simulink model "NON_COHERENT_RECEIVER"  (R2021b)
settings: Solver=VariableStepAuto  StartTime=0.0  StopTime=inf  RelTol=1e-3
libraries: simulink x3, dspsigops x3, dsparch4 x2, commfilt2 x2, dspsrcs4 x1
settings Model: Creator=caccolillo  LastModifiedBy=caccolillo

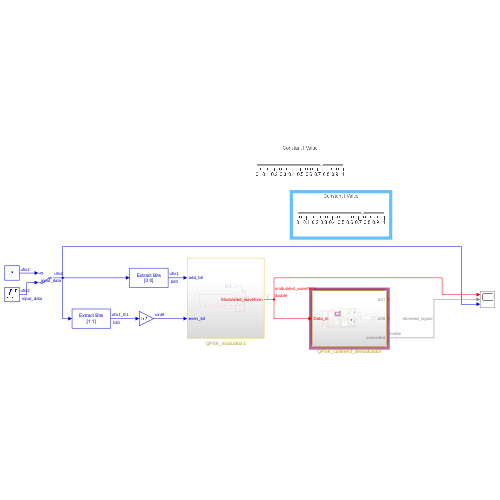
[thumbnail: Simulink's stored preview of the top-level diagram]
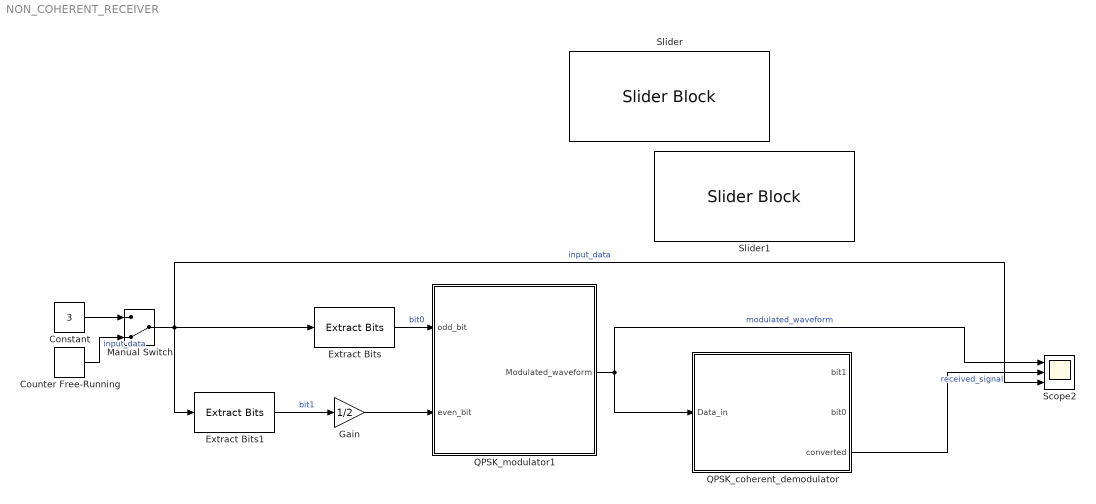
== system NON_COHERENT_RECEIVER ==
  Constant : Constant  Value=3  OutDataTypeStr=fixdt(0,2)  SampleTime=1/20000
  Counter Free-Running : simulink/Sources/Counter Free-Running  NumBits=2  tsamp=1/20000
  Extract Bits : simulink/Logic and Bit Operations/Extract Bits  bitsToExtract=Range of bits  numBits=8  bitIdxRange=[0 0]  outScalingMode=Preserve fixed-point scaling
  Extract Bits1 : simulink/Logic and Bit Operations/Extract Bits  bitsToExtract=Range of bits  numBits=8  bitIdxRange=[1 1]  outScalingMode=Preserve fixed-point scaling
  Gain : Gain  Gain=1/2
  Manual Switch : ManualSwitch  CurrentSetting=0
  QPSK_coherent_demodulator : Subsystem
  QPSK_modulator1 : Subsystem
  Scope2 : Scope  NumInputPorts=3
  Slider : SliderBlock  ScaleMax=1
  Slider1 : SliderBlock  ScaleMax=1
  wires:
  QPSK_modulator1/1(Modulated_waveform) -> QPSK_coherent_demodulator/1(Data_in), Scope2/1  "modulated_waveform"
  Manual Switch/1 -> Extract Bits1/1, Scope2/3, Extract Bits/1  "input_data"
  Gain/1 -> QPSK_modulator1/2(even_bit)
  Constant/1 -> Manual Switch/1
  Extract Bits1/1 -> Gain/1  "bit1"
  QPSK_coherent_demodulator/3(converted) -> Scope2/2  "received_signal"
  Counter Free-Running/1 -> Manual Switch/2  "input_data"
  Extract Bits/1 -> QPSK_modulator1/1(odd_bit)  "bit0"

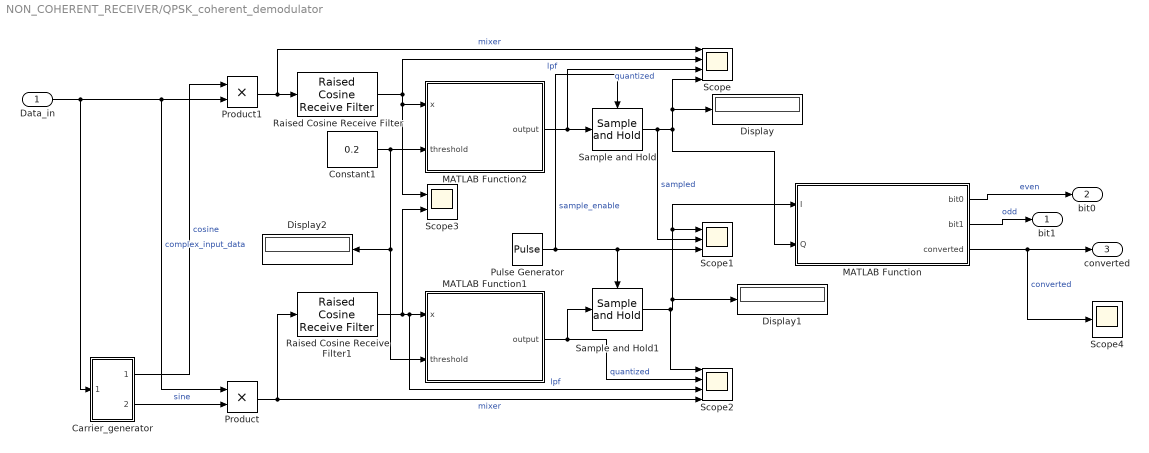
== system NON_COHERENT_RECEIVER/QPSK_coherent_demodulator ==
  Data_in : Inport
  Carrier_generator : Subsystem
  Constant1 : Constant  Value=0.2
  Display : Display
  Display1 : Display
  Display2 : Display
  MATLAB Function : MATLAB Function  TreatAsAtomicUnit=on
  MATLAB Function1 : MATLAB Function  TreatAsAtomicUnit=on
  MATLAB Function2 : MATLAB Function  TreatAsAtomicUnit=on
  Product : Product
  Product1 : Product
  Pulse Generator : DiscretePulseGenerator  PulseType=Time based  Period=1/20000  PulseWidth=5
  Raised Cosine Receive Filter : commfilt2/Raised Cosine Receive Filter  filtType=Square root  R=0.2  filtSpan=10  N=10  downFactor=2  downOffset=0  filterGain=1  RateOptions=Allow multirate processing  framing=Mute  checkCoeff=off  variableName=rcRxFilt  currentFiltSpan=10  D=5  inputOffset=0  sampMode=Mute  saveAsFlag=0  rateMode=Downsampling  checkGain=Normalized  launchFVT=on  roundingMode=Floor  overflowMode=off  coeffDataTypeStr=Inherit: Same word length as input  coeffMin=[]  coeffMax=[]  coeffLastDataTypeStr=Inherit: Same word length as input  accumDataTypeStr=Inherit: Same as product output  accumLastDataTypeStr=Inherit: Same as product output  outputDataTypeStr=Inherit: Same as accumulator  outputMin=[]  outputMax=[]  outputLastDataTypeStr=Inherit: Same as accumulator
  Raised Cosine Receive Filter1 : commfilt2/Raised Cosine Receive Filter  filtType=Square root  R=0.2  filtSpan=10  N=10  downFactor=2  downOffset=0  filterGain=1  RateOptions=Allow multirate processing  framing=Mute  checkCoeff=off  variableName=rcRxFilt1  currentFiltSpan=10  D=5  inputOffset=0  sampMode=Mute  saveAsFlag=0  rateMode=Downsampling  checkGain=Normalized  launchFVT=on  roundingMode=Floor  overflowMode=off  coeffDataTypeStr=Inherit: Same word length as input  coeffMin=[]  coeffMax=[]  coeffLastDataTypeStr=Inherit: Same word length as input  accumDataTypeStr=Inherit: Same as product output  accumLastDataTypeStr=Inherit: Same as product output  outputDataTypeStr=Inherit: Same as accumulator  outputMin=[]  outputMax=[]  outputLastDataTypeStr=Inherit: Same as accumulator
  Sample and Hold : dspsigops/Sample and Hold  trig=Rising edge  initCond=0  latchinput=off
  Sample and Hold1 : dspsigops/Sample and Hold  trig=Rising edge  initCond=0  latchinput=off
  Scope : Scope  NumInputPorts=4
  Scope1 : Scope  NumInputPorts=3
  Scope2 : Scope  NumInputPorts=4
  Scope3 : Scope  NumInputPorts=2
  Scope4 : Scope
  bit1 : Outport
  bit0 : Outport  Port=2
  converted : Outport  Port=3
  wires:
  Data_in/1 -> Carrier_generator/1(Modulated_signal), Product/1, Product1/2  "complex_input_data"
  Product1/1 -> Raised Cosine Receive Filter/1, Scope/1  "mixer"
  Raised Cosine Receive Filter/1 -> MATLAB Function2/1(x), Scope3/1, Scope/2  "lpf"
  Product/1 -> Raised Cosine Receive Filter1/1, Scope2/4  "mixer"
  Pulse Generator/1 -> Sample and Hold1/Trigger, Scope1/3, Sample and Hold/Trigger  "sample_enable"
  MATLAB Function1/1(output) -> Scope2/2, Sample and Hold1/1  "quantized"
  Sample and Hold/1 -> MATLAB Function/2(Q), Scope/4, Display/1, Scope1/2  "sampled"
  MATLAB Function2/1(output) -> Scope/3, Sample and Hold/1  "quantized"
  Carrier_generator/2(sine) -> Product/2  "sine"
  Sample and Hold1/1 -> Display1/1, MATLAB Function/1(I), Scope1/1, Scope2/1
  Carrier_generator/1(cosine) -> Product1/1  "cosine"
  Raised Cosine Receive Filter1/1 -> Scope2/3, MATLAB Function1/1(x), Scope3/2  "lpf"
  MATLAB Function/1(bit0) -> bit0/1  "even"
  MATLAB Function/2(bit1) -> bit1/1  "odd"
  MATLAB Function/3(converted) -> converted/1, Scope4/1  "converted"
  Constant1/1 -> Display2/1, MATLAB Function1/2(threshold), MATLAB Function2/2(threshold)

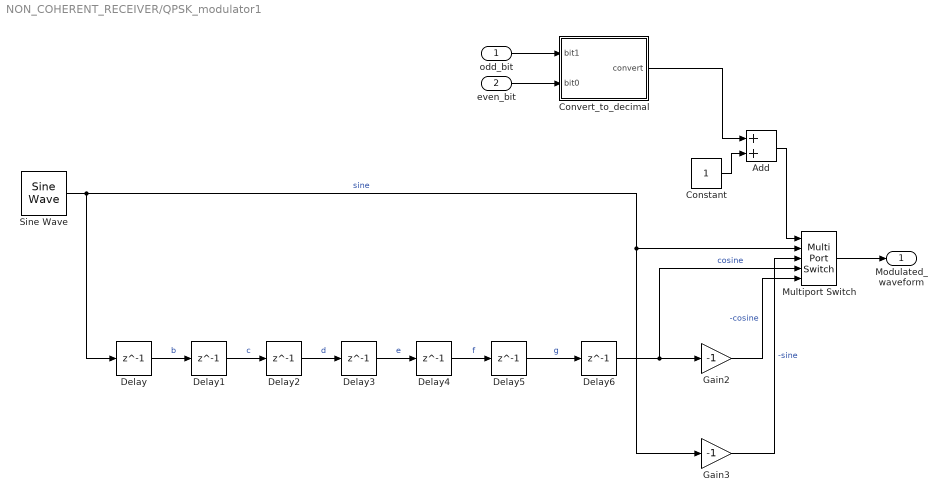
== system NON_COHERENT_RECEIVER/QPSK_modulator1 ==
  odd_bit : Inport
  even_bit : Inport  Port=2
  Add : Sum
  Constant : Constant
  Convert_to_decimal : Subsystem
  Delay{,1..6} (7 alike) : Delay  DelayLength=1  InitialCondition=0
  Gain2 : Gain  Gain=-1
  Gain3 : Gain  Gain=-1
  Multiport Switch : MultiPortSwitch  Inputs=4
  Sine Wave : dspsrcs4/Sine Wave  Amplitude=1  Frequency=20000  Phase=0  SampleMode=Discrete  OutComplex=Real  CompMethod=Table lookup  TableSize=Speed  SampleTime=1/200000  SamplesPerFrame=1  ResetState=Restart at time zero  OutputFrames=off  dataType=double  wordLen=16  udDataType=sfix(16)  fracBitsMode=Best precision  numFracBits=15  OutDataTypeStr=double  LastOutDataTypeStr=double
  Modulated_waveform : Outport
  wires:
  Gain3/1 -> Multiport Switch/3  "-sine"
  Sine Wave/1 -> Multiport Switch/2, Gain3/1, Delay/1  "sine"
  Delay/1 -> Delay1/1  "b"
  Delay1/1 -> Delay2/1  "c"
  Delay6/1 -> Multiport Switch/4, Gain2/1  "cosine"
  Multiport Switch/1 -> Modulated_waveform/1
  Delay3/1 -> Delay4/1  "e"
  Gain2/1 -> Multiport Switch/5  "-cosine"
  Delay4/1 -> Delay5/1  "f"
  odd_bit/1 -> Convert_to_decimal/1(bit1)
  Delay2/1 -> Delay3/1  "d"
  Convert_to_decimal/1(convert) -> Add/1
  Constant/1 -> Add/2
  Add/1 -> Multiport Switch/1
  even_bit/1 -> Convert_to_decimal/2(bit0)
  Delay5/1 -> Delay6/1  "g"

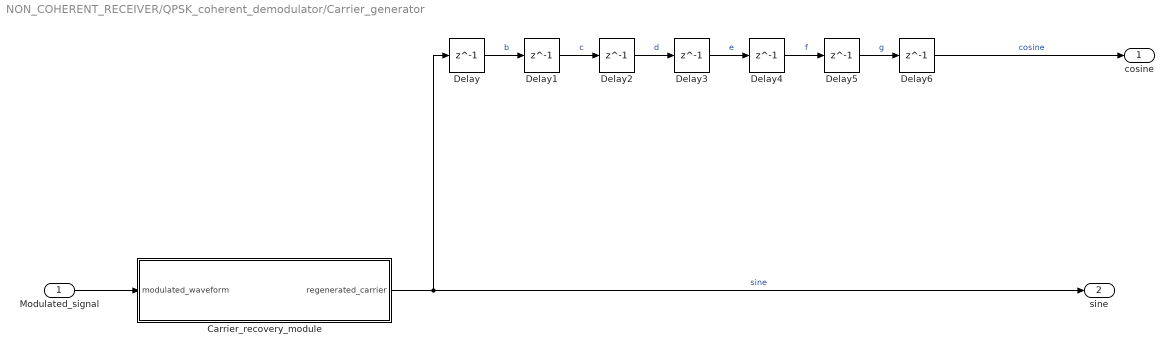
== system NON_COHERENT_RECEIVER/QPSK_coherent_demodulator/Carrier_generator ==
  Modulated_signal : Inport
  Carrier_recovery_module : Subsystem
  Delay{,1..6} (7 alike) : Delay  DelayLength=1  InitialCondition=0
  cosine : Outport
  sine : Outport  Port=2
  wires:
  Delay1/1 -> Delay2/1  "c"
  Delay5/1 -> Delay6/1  "g"
  Delay2/1 -> Delay3/1  "d"
  Carrier_recovery_module/1(regenerated_carrier) -> Delay/1, sine/1  "sine"
  Delay6/1 -> cosine/1  "cosine"
  Delay3/1 -> Delay4/1  "e"
  Delay/1 -> Delay1/1  "b"
  Delay4/1 -> Delay5/1  "f"
  Modulated_signal/1 -> Carrier_recovery_module/1(modulated_waveform)

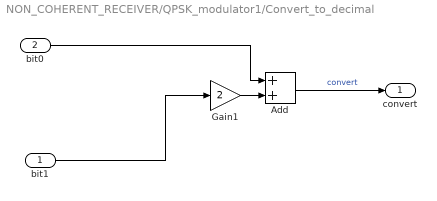
== system NON_COHERENT_RECEIVER/QPSK_modulator1/Convert_to_decimal ==
  bit1 : Inport
  bit0 : Inport  Port=2
  Add : Sum
  Gain1 : Gain  Gain=2
  convert : Outport
  wires:
  bit1/1 -> Gain1/1
  bit0/1 -> Add/1
  Add/1 -> convert/1  "convert"
  Gain1/1 -> Add/2

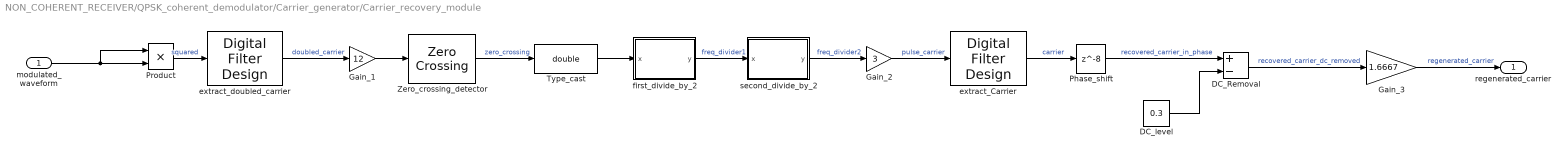
== system NON_COHERENT_RECEIVER/QPSK_coherent_demodulator/Carrier_generator/Carrier_recovery_module ==
  modulated_waveform : Inport
  DC_Removal : Sum  Inputs=+-
  DC_level : Constant  Value=0.3
  Gain_1 : Gain  Gain=12
  Gain_2 : Gain  Gain=3
  Gain_3 : Gain  Gain=1.6667
  Phase_shift : Delay  DelayLength=8
  Product : Product
  Type_cast : DataTypeConversion  OutDataTypeStr=double
  Zero_crossing_detector : dspsigops/Zero Crossing  InputProcessing=Columns as channels (frame based)
      settings: SourceProductBaseCode=DS
  extract_Carrier : dsparch4/Digital Filter Design  mwdsp_browser_bugfix_var=off
  extract_doubled_carrier : dsparch4/Digital Filter Design  mwdsp_browser_bugfix_var=off
  first_divide_by_2 : MATLAB Function  TreatAsAtomicUnit=on
  second_divide_by_2 : MATLAB Function  TreatAsAtomicUnit=on
  regenerated_carrier : Outport
  wires:
  modulated_waveform/1 -> Product/1, Product/2
  DC_level/1 -> DC_Removal/2
  Gain_3/1 -> regenerated_carrier/1  "regenerated_carrier"
  Phase_shift/1 -> DC_Removal/1  "recovered_carrier_in_phase"
  DC_Removal/1 -> Gain_3/1  "recovered_carrier_dc_removed"
  Product/1 -> extract_doubled_carrier/1  "squared"
  extract_doubled_carrier/1 -> Gain_1/1  "doubled_carrier"
  Gain_2/1 -> extract_Carrier/1  "pulse_carrier"
  second_divide_by_2/1(y) -> Gain_2/1  "freq_divider2"
  first_divide_by_2/1(y) -> second_divide_by_2/1(x)  "freq_divider1"
  Gain_1/1 -> Zero_crossing_detector/1
  Type_cast/1 -> first_divide_by_2/1(x)
  extract_Carrier/1 -> Phase_shift/1  "carrier"
  Zero_crossing_detector/1 -> Type_cast/1  "zero_crossing"

== matlab function NON_COHERENT_RECEIVER/QPSK_coherent_demodulator/MATLAB Function1 ==
  data: x input; output output; threshold input
function output = discretize_input(x,threshold)
    if x > threshold
        output = 1;
    else
        output = 0;
    end
end

== matlab function NON_COHERENT_RECEIVER/QPSK_coherent_demodulator/MATLAB Function2 ==
  data: x input; output output; threshold input
function output = discretize_input(x,threshold)
    if x > threshold
        output = 1;
    else
        output = 0;
    end
end

== matlab function NON_COHERENT_RECEIVER/QPSK_coherent_demodulator/Carrier_generator/Carrier_recovery_module/first_divide_by_2 ==
  data: x input; y output
function y = freqDivider(x)
% freqDivider  Frequency divider using persistent 2-sample input buffer
%
%   y = freqDivider(x) processes a single input sample x (scalar), and
%   returns a scalar output y, which goes high on every second rising edge.
%
%   This function is stateful and maintains internal buffer and edge counter
%   across calls using persistent variables.

    % Declare persistent variables
    persistent buf riseCount

    % Initialize persistent variables on first call
    if isempty(buf)
        buf = [0, 0];      % input buffer: [x(i-2), x(i-1)]
        riseCount = 0;     % rising edge counter
    end

    % Shift input buffer
    buf = [buf(2), x];

    % Default output
    y = 0;

    % Detect rising edge: x(i-1) <= 0 and x(i) > 0
    if buf(1) <= 0 && buf(2) > 0
        riseCount = riseCount + 1;

        if mod(riseCount, 2) == 0
            y = 1;  % Output high on every 2nd rising edge
        end
    end
end

== matlab function NON_COHERENT_RECEIVER/QPSK_coherent_demodulator/MATLAB Function ==
  data: bit0 output; I input; bit1 output; Q input; converted output
function [bit0, bit1,converted] = qpsk_demod_scalar(I, Q)
%QPSK_DEMOD_SCALAR Demodulates one QPSK symbol (scalar I/Q) into two bits.
% Inputs:
%   I - In-phase component (scalar)
%   Q - Quadrature component (scalar)
% Outputs:
%   bit1 - First bit (MSB)
%   bit2 - Second bit (LSB)

    % QPSK Gray demapping
    if I == 1 && Q == 1
        bit0 = 0; bit1 = 0;
        converted = 0;
    elseif I == 0 && Q == 1
        bit0 = 0; bit1 = 1;
        converted = 1;
    elseif I == 0 && Q == 0
        bit0 = 0; bit1 = 1;
        converted = 2;
    elseif I == 1 && Q == 0
        bit0 = 1; bit1 = 1;
        converted = 3;
    else
        % Edge case: I or Q == 0 (treat as 0)
        bit0 = 0;
        bit1 = 0;
        converted = 0;
    end
end

== matlab function NON_COHERENT_RECEIVER/QPSK_coherent_demodulator/Carrier_generator/Carrier_recovery_module/second_divide_by_2 ==
  data: x input; y output
function y = freqDivider(x)
% freqDivider  Frequency divider using persistent 2-sample input buffer
%
%   y = freqDivider(x) processes a single input sample x (scalar), and
%   returns a scalar output y, which goes high on every second rising edge.
%
%   This function is stateful and maintains internal buffer and edge counter
%   across calls using persistent variables.

    % Declare persistent variables
    persistent buf riseCount

    % Initialize persistent variables on first call
    if isempty(buf)
        buf = [0, 0];      % input buffer: [x(i-2), x(i-1)]
        riseCount = 0;     % rising edge counter
    end

    % Shift input buffer
    buf = [buf(2), x];

    % Default output
    y = 0;

    % Detect rising edge: x(i-1) <= 0 and x(i) > 0
    if buf(1) <= 0 && buf(2) > 0
        riseCount = riseCount + 1;

        if mod(riseCount, 2) == 0
            y = 1;  % Output high on every 2nd rising edge
        end
    end
end
